simulink model "infinite"  (R2018a)
settings: Solver=VariableStepAuto  StartTime=0.0  StopTime=10.0  RelTol=1e-3
settings Model: Creator=BEAR  LastModifiedBy=BEAR

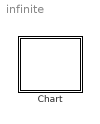
== system infinite ==
  Chart : Stateflow chart  TreatAsAtomicUnit=on

== stateflow chart infinite/Chart ==
  state A
  state B
  (default) -> A
  A -> B : {e}/{e}
  events: e local FUNCTION_CALL_EVENT
